simulink model "plantChange_CA3_model"  (R2023b)
settings: Solver=VariableStepAuto  StartTime=0.0  StopTime=200  RelTol=1e-3
values from neighbouring files (symbols this model uses):
  b = [0;1]    [CA3_param.m]
  C = 1    [CA3_param.m]
  Gamma = [100 0; 0 100]    [CA3_param.m]
  gamma = 1000    [CA3_param.m]
  K = 6.2    [CA3_param.m]
  K2 = 4.5    [CA3_param.m]
  k_theta = mdl1.Coefficients{1,1}    [CA3_param.m]
  P = lyap(Am', Q)    [CA3_param.m]
  tau = 0.25    [CA3_param.m]
  tau2 = 0.45    [CA3_param.m]
  w = 10    [CA3_param.m]
settings Model: Creator=jiang  LastModifiedBy=99551
settings DebuggingCC: UnconnectedInputMsg=warning  UnconnectedOutputMsg=warning  UnconnectedLineMsg=warning
settings ModelReferenceCC: EnableRefExpFcnMdlSchedulingChecks=on
settings RTWCC: DLArmComputeVersion=19.05

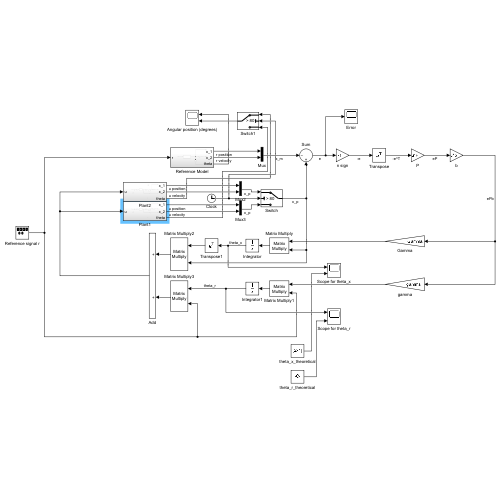
[thumbnail: Simulink's stored preview of the top-level diagram]
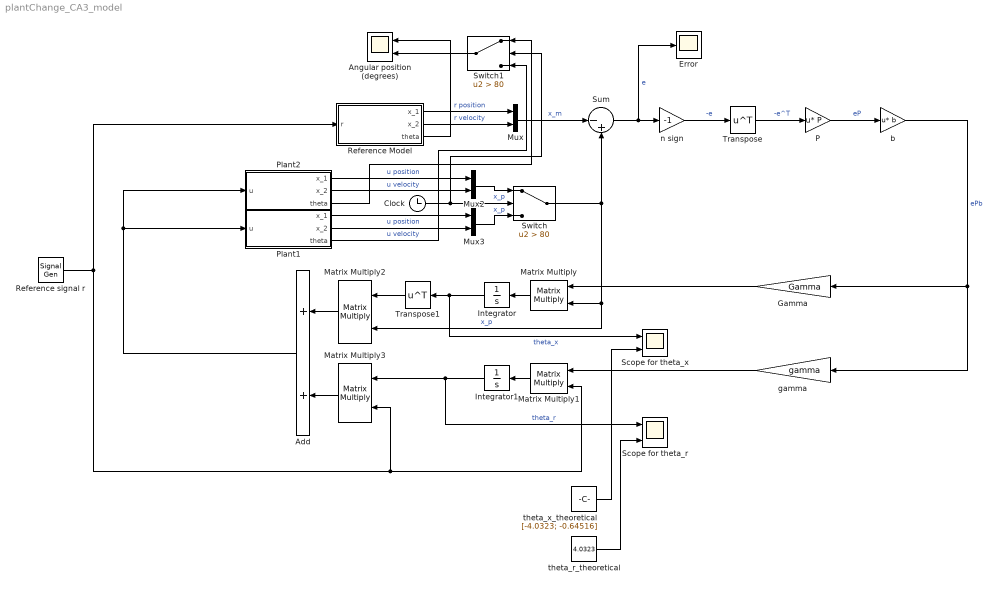
== system plantChange_CA3_model ==
  Add : Sum
  Angular position (degrees) : Scope  NumInputPorts=2
  Clock : Clock
  Error : Scope
  Gamma : Gain  Gain=Gamma
  Integrator : Integrator
  Integrator1 : Integrator
  Matrix Multiply{,1..3} (4 alike) : Product  Multiplication=Matrix(*)
  Mux : Mux  Inputs=2
  Mux2 : Mux  Inputs=2
  Mux3 : Mux  Inputs=2
  P : Gain  Gain=P  Multiplication=Matrix(u*K)
  Plant1 : Subsystem
  Plant2 : Subsystem
  Reference Model : Subsystem
  Reference signal r : SignalGenerator  WaveForm=square  Frequency=0.05
  Scope for theta_r : Scope  NumInputPorts=2
  Scope for theta_x : Scope  NumInputPorts=2
  Sum : Sum  Inputs=|-+
  Switch : Switch  Criteria=u2 > Threshold  Threshold=80  SaturateOnIntegerOverflow=off  InputSameDT=off
  Switch1 : Switch  Criteria=u2 > Threshold  Threshold=80  SaturateOnIntegerOverflow=off  InputSameDT=off
  Transpose : Math  Operator=transpose
  Transpose1 : Math  Operator=transpose
  b : Gain  Gain=b  Multiplication=Matrix(u*K)
  gamma : Gain  Gain=gamma
  n sign : Gain  Gain=-1
  theta_r_theoretical : Constant  Value=4.0323
  theta_x_theoretical : Constant  Value=[-4.0323; -0.64516]
  wires:
  Mux/1 -> Sum/1  "x_m"
  Switch/1 -> Matrix Multiply2/2, Matrix Multiply/2, Sum/2  "x_p"
  Sum/1 -> Error/1, n sign/1  "e"
  n sign/1 -> Transpose/1  "-e"
  Transpose/1 -> P/1  "-e^T"
  P/1 -> b/1  "eP"
  b/1 -> gamma/1, Gamma/1  "ePb"
  Gamma/1 -> Matrix Multiply/1
  gamma/1 -> Matrix Multiply1/1
  Matrix Multiply/1 -> Integrator/1
  Matrix Multiply1/1 -> Integrator1/1
  Integrator/1 -> Scope for theta_x/1, Transpose1/1  "theta_x"
  Transpose1/1 -> Matrix Multiply2/1
  Integrator1/1 -> Matrix Multiply3/1, Scope for theta_r/1  "theta_r"
  Matrix Multiply2/1 -> Add/1
  Matrix Multiply3/1 -> Add/2
  Reference Model/1(x_1) -> Mux/1  "r position"
  Reference Model/2(x_2) -> Mux/2  "r velocity"
  Reference Model/3(theta) -> Angular position (degrees)/1
  Add/1 -> Plant2/1(u), Plant1/1(u)
  theta_x_theoretical/1 -> Scope for theta_x/2
  theta_r_theoretical/1 -> Scope for theta_r/2
  Plant2/2(x_2) -> Mux2/2  "u velocity"
  Plant2/1(x_1) -> Mux2/1  "u position"
  Plant1/1(x_1) -> Mux3/1  "u position"
  Plant1/2(x_2) -> Mux3/2  "u velocity"
  Mux2/1 -> Switch/1  "x_p"
  Mux3/1 -> Switch/3  "x_p"
  Clock/1 -> Switch1/2, Switch/2
  Switch1/1 -> Angular position (degrees)/2
  Plant2/3(theta) -> Switch1/1
  Plant1/3(theta) -> Switch1/3
  Reference signal r/1 -> Matrix Multiply3/2, Matrix Multiply1/2, Reference Model/1(r)

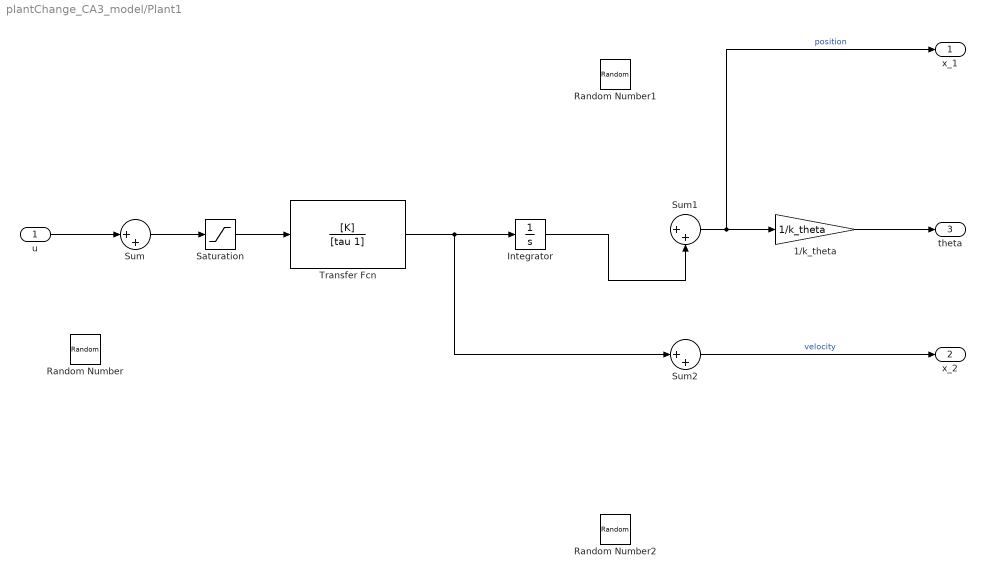
== system plantChange_CA3_model/Plant1 ==
  u : Inport
  1/k_theta : Gain  Gain=1/k_theta
  Integrator : Integrator
  Random Number : RandomNumber  Variance=0.1  SampleTime=0.01
  Random Number1 : RandomNumber  Variance=0.0001  SampleTime=0.01
  Random Number2 : RandomNumber  Variance=0.0001  SampleTime=0.01
  Saturation : Saturate  UpperLimit=5  LowerLimit=-5
  Sum : Sum  Inputs=|++
  Sum1 : Sum  Inputs=|++
  Sum2 : Sum  Inputs=|++
  Transfer Fcn : TransferFcn  Numerator=[K]  Denominator=[tau 1]
  x_1 : Outport
  x_2 : Outport  Port=2
  theta : Outport  Port=3
  wires:
  Sum/1 -> Saturation/1
  u/1 -> Sum/1
  Saturation/1 -> Transfer Fcn/1
  Transfer Fcn/1 -> Integrator/1, Sum2/1
  Integrator/1 -> Sum1/2
  Sum1/1 -> x_1/1, 1/k_theta/1  "position"
  Sum2/1 -> x_2/1  "velocity"
  1/k_theta/1 -> theta/1

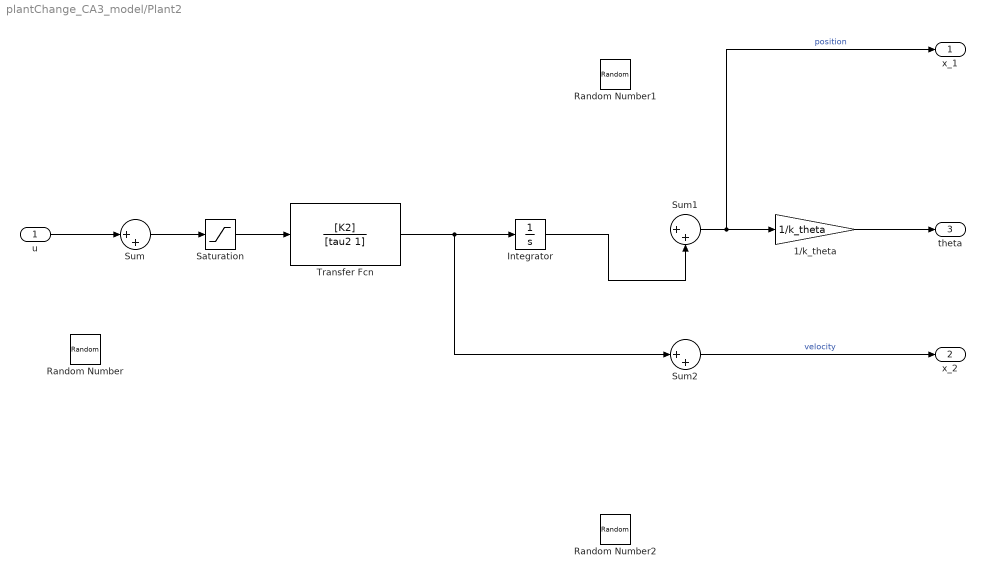
== system plantChange_CA3_model/Plant2 ==
  u : Inport
  1/k_theta : Gain  Gain=1/k_theta
  Integrator : Integrator
  Random Number : RandomNumber  Variance=0.1  SampleTime=0.01
  Random Number1 : RandomNumber  Variance=0.0001  SampleTime=0.01
  Random Number2 : RandomNumber  Variance=0.0001  SampleTime=0.01
  Saturation : Saturate  UpperLimit=5  LowerLimit=-5
  Sum : Sum  Inputs=|++
  Sum1 : Sum  Inputs=|++
  Sum2 : Sum  Inputs=|++
  Transfer Fcn : TransferFcn  Numerator=[K2]  Denominator=[tau2 1]
  x_1 : Outport
  x_2 : Outport  Port=2
  theta : Outport  Port=3
  wires:
  Sum/1 -> Saturation/1
  u/1 -> Sum/1
  Saturation/1 -> Transfer Fcn/1
  Transfer Fcn/1 -> Integrator/1, Sum2/1
  Integrator/1 -> Sum1/2
  Sum1/1 -> x_1/1, 1/k_theta/1  "position"
  Sum2/1 -> x_2/1  "velocity"
  1/k_theta/1 -> theta/1

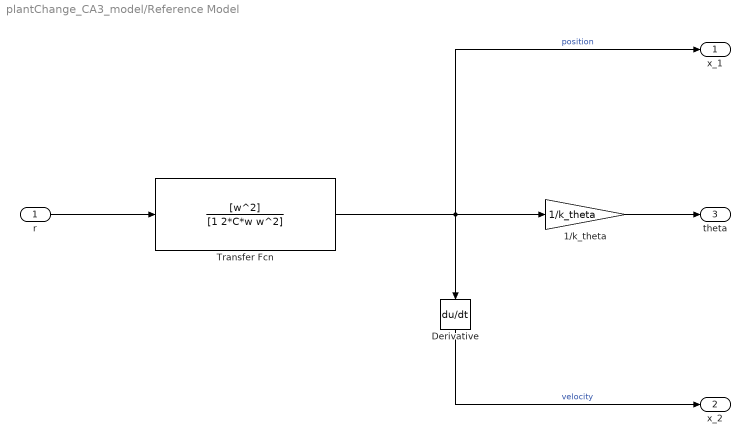
== system plantChange_CA3_model/Reference Model ==
  r : Inport
  1/k_theta : Gain  Gain=1/k_theta
  Derivative : Derivative
  Transfer Fcn : TransferFcn  Numerator=[w^2]  Denominator=[1 2*C*w w^2]
  x_1 : Outport
  x_2 : Outport  Port=2
  theta : Outport  Port=3
  wires:
  r/1 -> Transfer Fcn/1
  Transfer Fcn/1 -> x_1/1, 1/k_theta/1, Derivative/1  "position"
  Derivative/1 -> x_2/1  "velocity"
  1/k_theta/1 -> theta/1
